simulink model "array_doubleRx"  (R2019b)
settings: Solver=VariableStepAuto  StartTime=0.0  StopTime=0.0005  RelTol=1e-3
libraries: fl_lib x109, nesl_utility x70, ee_lib x35, powerlib_meascontrol x11
settings Model: Creator=LRF  LastModifiedBy=LRF

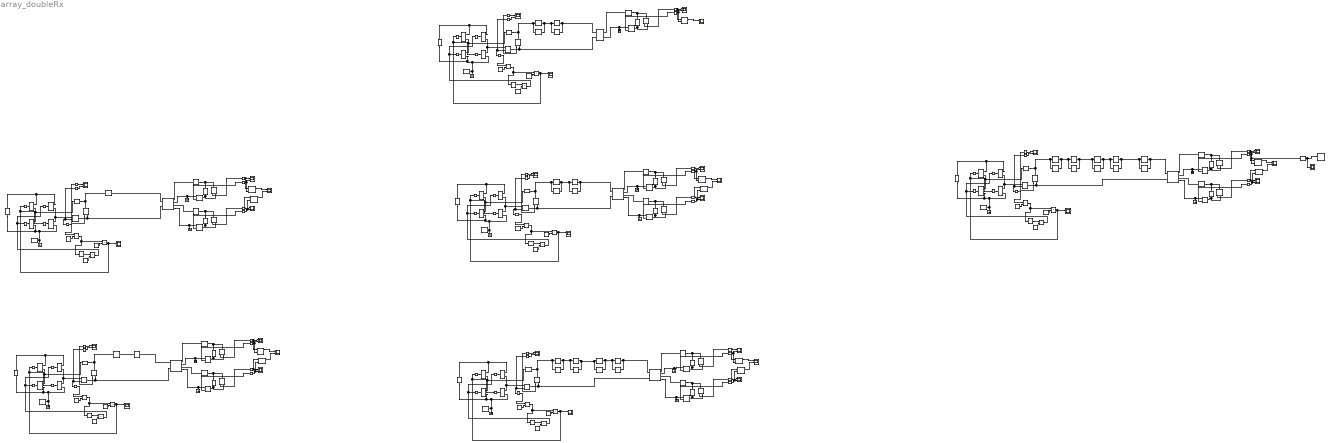
== system array_doubleRx ==
  (2/a-1)Ca{,1..12} (13 alike) : fl_lib/Electrical/Electrical Elements/Capacitor  c=379 pF  r=1e-6 Ohm  g=0 1/Ohm  i_specify=off  i_priority=None  i=0 A  i_nominal_specify=off  i_nominal_unit=A  i_nominal_value=1  v_specify=off  v_priority=None  v=0 V  v_nominal_specify=off  v_nominal_unit=V  v_nominal_value=1  vc_specify=off  vc_priority=High  vc=0 V  vc_nominal_specify=off  vc_nominal_unit=V  vc_nominal_value=1
  Ca{,1..15} (16 alike) : fl_lib/Electrical/Electrical Elements/Capacitor  c=1517 pF  r=1e-6 Ohm  g=0 1/Ohm  i_specify=off  i_priority=None  i=0 A  i_nominal_specify=off  i_nominal_unit=A  i_nominal_value=1  v_specify=off  v_priority=None  v=0 V  v_nominal_specify=off  v_nominal_unit=V  v_nominal_value=1  vc_specify=off  vc_priority=High  vc=0 V  vc_nominal_specify=off  vc_nominal_unit=V  vc_nominal_value=1
  Capacitor{1..10,12} (11 alike) : fl_lib/Electrical/Electrical Elements/Capacitor  c=1013 pF  r=1e-6 Ohm  g=0 1/Ohm  i_specify=off  i_priority=None  i=0 A  i_nominal_specify=off  i_nominal_unit=A  i_nominal_value=1  v_specify=off  v_priority=None  v=0 V  v_nominal_specify=off  v_nominal_unit=V  v_nominal_value=1  vc_specify=off  vc_priority=High  vc=0 V  vc_nominal_specify=off  vc_nominal_unit=V  vc_nominal_value=1
  Constant{,2,6,9,14..15} (6 alike) : Constant  Value=0
  Constant{1,3..5,7..8,10..13,16..17} (12 alike) : Constant  Value=12
  Current Sensor{,1..15,17} (17 alike) : fl_lib/Electrical/Electrical Sensors/Current Sensor
  Electrical Reference{,1..15,17} (17 alike) : fl_lib/Electrical/Electrical Elements/Electrical Reference
  GT{,1..5} (6 alike) : RelationalOperator  Operator=>  OutDataTypeStr=boolean  RndMeth=Simplest
  Logical Operator{,1..5} (6 alike) : Logic  Operator=NOT  AllPortsSameDT=off  OutDataTypeStr=boolean
  MOSFET (Ideal, Switching){,1..23} (24 alike) : ee_lib/Semiconductors & Converters/MOSFET (Ideal, Switching)  Rds=0.01 Ohm  Goff=1e-6 1/Ohm  Vth=2 V  diode_param=1  diode_Vf=0.8 V  diode_Ron=0.001 Ohm  diode_Goff=1e-5 1/Ohm  diode_C=50e-9 F  diode_iRM=-235 A  diode_iF=300 A  diode_idot=-50 A/us  diode_trr_param=1  diode_trr_factor=3  diode_trr=15 us  diode_Qrr=1500 s*uA  thermal_loss_option=2  Voff=300 V  Tau=1e-4 s  Tj=[298.15, 398.15] K  Iout_scalar=600 A  Eon_scalar=22.86e-3 J  Eoff_scalar=17.14e-3 J  Von_scalar=2.7 V  Iout_data=[0, 10, 50, 100, 200, 400, 600] A  Eon_data=[0, .29, 1.43, 2.86, 5.71, 13.14, 22.86; 0, .57, 2.63, 5.14, 10.29, 20.57, 30.29] * 1e-3 J  Eoff_data=[0, .21, 1.07, 2.14, 4.29, 9.86, 17.14; 0, .43, 1.97, 3.86, 7.71, 15.43, 22.71] * 1e-3 J  Von_data=[0, 1.1, 1.3, 1.45, 1.75, 2.25, 2.7; 0, 1, 1.15, 1.35, 1.7, 2.35, 3] V
      settings: SourceProductName=Simscape Electrical
  Mutual Inductor : fl_lib/Electrical/Electrical Elements/Mutual Inductor  L1=106.94 uH  L2=100 uH  k=0.1  i1_specify=off  i1_priority=High  i1=0 A  i1_nominal_specify=off  i1_nominal_unit=A  i1_nominal_value=1  i2_specify=off  i2_priority=High  i2=0 A  i2_nominal_specify=off  i2_nominal_unit=A  i2_nominal_value=1  v1_specify=off  v1_priority=None  v1=0 V  v1_nominal_specify=off  v1_nominal_unit=V  v1_nominal_value=1  v2_specify=off  v2_priority=None  v2=0 V  v2_nominal_specify=off  v2_nominal_unit=V  v2_nominal_value=1
      settings: SourceProductName=Simscape  SourceProductBaseCode=SS  InternalSimscapePortConfiguration="{\"Bottom\":[],\"Left\":[{\"id\":\"p1\",\"label\":\"1+\",\"type\":\"foundation.electrical.electrical\"},{\"id\":\"n1\",\"label\":\"1-\",\"type\":\"foundation.electrical.electrical\"}],\"Right\":[{\"id\":\"p2\",\"label\":\"2+\",\"type\":\"foundation.electrical.electrical\"},{\"id\":\"n2\",\"label\":\"2-\",\"type\":\"foundation.electrical.electrical\"}],\"Top\":[]}"
  PS-Simulink Converter{,1..37,40..41} (40 alike) : nesl_utility/PS-Simulink Converter  PhysicalDomain=network_engine_domain  SubClassName=ps_output  LeftPortType=input  RightPortType=output  PseudoPeriodic=off  Frequencies=[]  Unit=inherit  AffineConversion=off
  Power (Phasor){,1..9,11} (11 alike) : powerlib_meascontrol/Measurements/Power (Phasor)
      settings: SourceProductName=Simscape Electrical  SourceProductBaseCode=PS
  Product{,1..11} (12 alike) : Product
  Resistor{,3,6,9,14..15} (6 alike) : fl_lib/Electrical/Electrical Elements/Resistor  R=0 Ohm  i_specify=off  i_priority=None  i=0 A  i_nominal_specify=off  i_nominal_unit=A  i_nominal_value=1  v_specify=off  v_priority=None  v=0 V  v_nominal_specify=off  v_nominal_unit=V  v_nominal_value=1
  Resistor{1..2,4..5,7..8,10..13,17} (11 alike) : fl_lib/Electrical/Electrical Elements/Resistor  R=15 Ohm  i_specify=off  i_priority=None  i=0 A  i_nominal_specify=off  i_nominal_unit=A  i_nominal_value=1  v_specify=off  v_priority=None  v=0 V  v_nominal_specify=off  v_nominal_unit=V  v_nominal_value=1
  Scope{,1..24,26..27,29..30} (29 alike) : Scope  NumInputPorts=2
  Scope28 : Scope
  Simulink-PS Converter{,1..23} (24 alike) : nesl_utility/Simulink-PS Converter  PhysicalDomain=network_engine_domain  SubClassName=ps_input  LeftPortType=input  RightPortType=output  PseudoPeriodic=off  Frequencies=[]  NoiseDistribution=none  NoiseParameters=[]  Unit=1  AffineConversion=off  FilteringAndDerivatives=provide  SimscapeFilterOrder=1  InputFilterTimeConstant=0.001  UdotUserProvided=0
  Solver Configuration{,1..5} (6 alike) : nesl_utility/Solver Configuration  PhysicalDomain=network_engine_domain  SubClassName=solver  LeftPortType=input  RightPortType=generic  Tones=[]  Harmonics=[]  SimulateNoise=off  Profile=off  UseLocalSampling=off  EnableSwitchedLinearOptims=on  FrequencyDomain=off  UseCCode=off  RelTol=0.001  AbsTol=1e-06  MinStep=1e-09  ToWorkspace=off  RevertToSquareIcSolve=off  NumHomotopyIterations=100  PhasorMode=off  PhasorModeNumHarmonics=1  DoDC=off  ResidualTolerance=1e-09  UseLocalSolver=off  LocalSolverChoice=NE_BACKWARD_EULER_ADVANCER  LocalSolverSampleTime=0.001  DoFixedCost=off  MaxNonlinIter=3  MaxModeIter=2  LinearAlgebra=auto  EquationFormulation=NE_TIME_EF  DelaysMemoryBudget=1024  AutomaticFiltering=on  FilteringTimeConstant=0.001  PartitionStorageMethod=AS_NEEDED  PartitionMemoryBudget=1024  PartitionMethod=ROBUST
  Spectrum Analyzer2 : SpectrumAnalyzer
  Three-Winding Mutual Inductor : ee_lib/Passive/Transformers/Three-Winding Mutual Inductor  L1=106.94 uH  L2=100 uH  L3=100 uH  K12=0.1  K13=0.1  K23=0  IC_given=1  IC1=0 A  IC2=0 A  IC3=0 A
      settings: SourceProductName=Simscape Electrical  SourceProductBaseCode=PS  InternalSimscapePortConfiguration="{\"Bottom\":[],\"Left\":[{\"id\":\"p1\",\"label\":\"1+\",\"type\":\"foundation.electrical.electrical\"},{\"id\":\"n1\",\"label\":\"1-\",\"type\":\"foundation.electrical.electrical\"}],\"Right\":[{\"id\":\"p2\",\"label\":\"2+\",\"type\":\"foundation.electrical.electrical\"},{\"id\":\"n2\",\"label\":\"2-\",\"type\":\"foundation.electrical.electrical\"},{\"id\":\"p3\",\"label\":\"3+\",\"type\":\"foundation.electrical.electrical\"},{\"id\":\"n3\",\"label\":\"3-\",\"type\":\"foundation.electrical.electrical\"}],\"Top\":[]}"
  Three-Winding Mutual Inductor1 : ee_lib/Passive/Transformers/Three-Winding Mutual Inductor  L1=66.79 uH  L2=100 uH  L3=100 uH  K12=0.1  K13=0.1  K23=0  IC_given=1  IC1=0 A  IC2=0 A  IC3=0 A
      settings: SourceProductName=Simscape Electrical  SourceProductBaseCode=PS  InternalSimscapePortConfiguration="{\"Bottom\":[],\"Left\":[{\"id\":\"p1\",\"label\":\"1+\",\"type\":\"foundation.electrical.electrical\"},{\"id\":\"n1\",\"label\":\"1-\",\"type\":\"foundation.electrical.electrical\"}],\"Right\":[{\"id\":\"p2\",\"label\":\"2+\",\"type\":\"foundation.electrical.electrical\"},{\"id\":\"n2\",\"label\":\"2-\",\"type\":\"foundation.electrical.electrical\"},{\"id\":\"p3\",\"label\":\"3+\",\"type\":\"foundation.electrical.electrical\"},{\"id\":\"n3\",\"label\":\"3-\",\"type\":\"foundation.electrical.electrical\"}],\"Top\":[]}"
  Three-Winding Mutual Inductor2 : ee_lib/Passive/Transformers/Three-Winding Mutual Inductor  L1=133.58 uH  L2=100 uH  L3=100 uH  K12=0.1  K13=0.1  K23=0  IC_given=1  IC1=0 A  IC2=0 A  IC3=0 A
      settings: SourceProductName=Simscape Electrical  SourceProductBaseCode=PS  InternalSimscapePortConfiguration="{\"Bottom\":[],\"Left\":[{\"id\":\"p1\",\"label\":\"1+\",\"type\":\"foundation.electrical.electrical\"},{\"id\":\"n1\",\"label\":\"1-\",\"type\":\"foundation.electrical.electrical\"}],\"Right\":[{\"id\":\"p2\",\"label\":\"2+\",\"type\":\"foundation.electrical.electrical\"},{\"id\":\"n2\",\"label\":\"2-\",\"type\":\"foundation.electrical.electrical\"},{\"id\":\"p3\",\"label\":\"3+\",\"type\":\"foundation.electrical.electrical\"},{\"id\":\"n3\",\"label\":\"3-\",\"type\":\"foundation.electrical.electrical\"}],\"Top\":[]}"
  Three-Winding Mutual Inductor3 : ee_lib/Passive/Transformers/Three-Winding Mutual Inductor  L1=213.88 uH  L2=100 uH  L3=100 uH  K12=0.1  K13=0.1  K23=0  IC_given=1  IC1=0 A  IC2=0 A  IC3=0 A
      settings: SourceProductName=Simscape Electrical  SourceProductBaseCode=PS  InternalSimscapePortConfiguration="{\"Bottom\":[],\"Left\":[{\"id\":\"p1\",\"label\":\"1+\",\"type\":\"foundation.electrical.electrical\"},{\"id\":\"n1\",\"label\":\"1-\",\"type\":\"foundation.electrical.electrical\"}],\"Right\":[{\"id\":\"p2\",\"label\":\"2+\",\"type\":\"foundation.electrical.electrical\"},{\"id\":\"n2\",\"label\":\"2-\",\"type\":\"foundation.electrical.electrical\"},{\"id\":\"p3\",\"label\":\"3+\",\"type\":\"foundation.electrical.electrical\"},{\"id\":\"n3\",\"label\":\"3-\",\"type\":\"foundation.electrical.electrical\"}],\"Top\":[]}"
  Three-Winding Mutual Inductor4 : ee_lib/Passive/Transformers/Three-Winding Mutual Inductor  L1=280.67 uH  L2=100 uH  L3=100 uH  K12=0.1  K13=0.1  K23=0  IC_given=1  IC1=0 A  IC2=0 A  IC3=0 A
      settings: SourceProductName=Simscape Electrical  SourceProductBaseCode=PS  InternalSimscapePortConfiguration="{\"Bottom\":[],\"Left\":[{\"id\":\"p1\",\"label\":\"1+\",\"type\":\"foundation.electrical.electrical\"},{\"id\":\"n1\",\"label\":\"1-\",\"type\":\"foundation.electrical.electrical\"}],\"Right\":[{\"id\":\"p2\",\"label\":\"2+\",\"type\":\"foundation.electrical.electrical\"},{\"id\":\"n2\",\"label\":\"2-\",\"type\":\"foundation.electrical.electrical\"},{\"id\":\"p3\",\"label\":\"3+\",\"type\":\"foundation.electrical.electrical\"},{\"id\":\"n3\",\"label\":\"3-\",\"type\":\"foundation.electrical.electrical\"}],\"Top\":[]}"
  Voltage Sensor{,1..14,16..17} (17 alike) : fl_lib/Electrical/Electrical Sensors/Voltage Sensor
  Voltage Source : ee_lib/Sources/Voltage Source  dc_voltage=15 V  ac_voltage=0 V  ac_shift=0 rad  ac_frequency=60 Hz  noise_mode=0  PSD=0 V^2/Hz  repeatability=1  auto_seed=3646982598  user_seed=0  sample_time=1e-3 s  i_specify=off  i_priority=None  i=0 A  i_nominal_specify=off  i_nominal_unit=A  i_nominal_value=1  v_specify=off  v_priority=None  v=0 V  v_nominal_specify=off  v_nominal_unit=V  v_nominal_value=1
      settings: SourceProductName=Simscape Electrical
  Voltage Source1 : ee_lib/Sources/Voltage Source  dc_voltage=15 V  ac_voltage=0 V  ac_shift=0 rad  ac_frequency=60 Hz  noise_mode=0  PSD=0 V^2/Hz  repeatability=1  auto_seed=508128604  user_seed=0  sample_time=1e-3 s  i_specify=off  i_priority=None  i=0 A  i_nominal_specify=off  i_nominal_unit=A  i_nominal_value=1  v_specify=off  v_priority=None  v=0 V  v_nominal_specify=off  v_nominal_unit=V  v_nominal_value=1
      settings: SourceProductName=Simscape Electrical
  Voltage Source2 : ee_lib/Sources/Voltage Source  dc_voltage=15 V  ac_voltage=0 V  ac_shift=0 rad  ac_frequency=60 Hz  noise_mode=0  PSD=0 V^2/Hz  repeatability=1  auto_seed=746822400  user_seed=0  sample_time=1e-3 s  i_specify=off  i_priority=None  i=0 A  i_nominal_specify=off  i_nominal_unit=A  i_nominal_value=1  v_specify=off  v_priority=None  v=0 V  v_nominal_specify=off  v_nominal_unit=V  v_nominal_value=1
      settings: SourceProductName=Simscape Electrical
  Voltage Source3 : ee_lib/Sources/Voltage Source  dc_voltage=15 V  ac_voltage=0 V  ac_shift=0 rad  ac_frequency=60 Hz  noise_mode=0  PSD=0 V^2/Hz  repeatability=1  auto_seed=3181899151  user_seed=0  sample_time=1e-3 s  i_specify=off  i_priority=None  i=0 A  i_nominal_specify=off  i_nominal_unit=A  i_nominal_value=1  v_specify=off  v_priority=None  v=0 V  v_nominal_specify=off  v_nominal_unit=V  v_nominal_value=1
      settings: SourceProductName=Simscape Electrical
  Voltage Source4 : ee_lib/Sources/Voltage Source  dc_voltage=15 V  ac_voltage=0 V  ac_shift=0 rad  ac_frequency=60 Hz  noise_mode=0  PSD=0 V^2/Hz  repeatability=1  auto_seed=170723637  user_seed=0  sample_time=1e-3 s  i_specify=off  i_priority=None  i=0 A  i_nominal_specify=off  i_nominal_unit=A  i_nominal_value=1  v_specify=off  v_priority=None  v=0 V  v_nominal_specify=off  v_nominal_unit=V  v_nominal_value=1
      settings: SourceProductName=Simscape Electrical
  Voltage Source5 : ee_lib/Sources/Voltage Source  dc_voltage=15 V  ac_voltage=0 V  ac_shift=0 rad  ac_frequency=60 Hz  noise_mode=0  PSD=0 V^2/Hz  repeatability=1  auto_seed=2586388248  user_seed=0  sample_time=1e-3 s  i_specify=off  i_priority=None  i=0 A  i_nominal_specify=off  i_nominal_unit=A  i_nominal_value=1  v_specify=off  v_priority=None  v=0 V  v_nominal_specify=off  v_nominal_unit=V  v_nominal_value=1
      settings: SourceProductName=Simscape Electrical
  Zero-Order Hold1 : ZeroOrderHold  SampleTime=1e-7
  wires:
  PS-Simulink Converter/1 -> Scope/1
  PS-Simulink Converter2/1 -> Scope/2
  PS-Simulink Converter1/1 -> GT/1
  Constant/1 -> GT/2
  GT/1 -> Logical Operator/1, Product/1
  Product/1 -> Simulink-PS Converter3/1, Simulink-PS Converter1/1, Scope1/1
  Constant3/1 -> Product/2
  Logical Operator/1 -> Product1/1
  Constant1/1 -> Product1/2
  Product1/1 -> Simulink-PS Converter2/1, Simulink-PS Converter/1
  PS-Simulink Converter4/1 -> Power (Phasor)/2, Scope2/2
  PS-Simulink Converter3/1 -> Power (Phasor)/1, Scope2/1
  PS-Simulink Converter6/1 -> Power (Phasor)1/2, Scope3/2
  PS-Simulink Converter5/1 -> Power (Phasor)1/1, Scope3/1
  Power (Phasor)/1 -> Scope4/2
  Power (Phasor)1/1 -> Scope4/1
  PS-Simulink Converter7/1 -> Scope5/1
  PS-Simulink Converter9/1 -> Scope5/2
  PS-Simulink Converter8/1 -> GT1/1
  PS-Simulink Converter13/1 -> Power (Phasor)3/2, Scope8/2
  Power (Phasor)2/1 -> Scope9/2
  GT1/1 -> Logical Operator1/1, Product2/1
  PS-Simulink Converter10/1 -> Power (Phasor)2/1, Scope7/1
  Product2/1 -> Simulink-PS Converter7/1, Simulink-PS Converter5/1, Scope6/1
  Logical Operator1/1 -> Product3/1
  Product3/1 -> Simulink-PS Converter6/1, Simulink-PS Converter4/1
  Constant2/1 -> GT1/2
  PS-Simulink Converter11/1 -> Power (Phasor)2/2, Scope7/2
  Power (Phasor)3/1 -> Scope9/1
  Constant5/1 -> Product2/2
  Constant4/1 -> Product3/2
  PS-Simulink Converter12/1 -> Power (Phasor)3/1, Scope8/1
  Product5/1 -> Simulink-PS Converter10/1, Simulink-PS Converter8/1
  Logical Operator2/1 -> Product5/1
  GT2/1 -> Logical Operator2/1, Product4/1
  PS-Simulink Converter18/1 -> Scope10/1
  PS-Simulink Converter17/1 -> Power (Phasor)5/2, Scope13/2
  PS-Simulink Converter20/1 -> Scope10/2
  PS-Simulink Converter19/1 -> GT2/1
  Constant8/1 -> Product4/2
  Product4/1 -> Simulink-PS Converter11/1, Simulink-PS Converter9/1, Scope11/1
  PS-Simulink Converter16/1 -> Power (Phasor)5/1, Scope13/1
  PS-Simulink Converter15/1 -> Power (Phasor)4/2, Scope12/2
  PS-Simulink Converter14/1 -> Power (Phasor)4/1, Scope12/1
  Constant6/1 -> GT2/2
  Constant7/1 -> Product5/2
  Power (Phasor)5/1 -> Scope14/1
  Power (Phasor)4/1 -> Scope14/2
  PS-Simulink Converter21/1 -> Scope15/1
  PS-Simulink Converter23/1 -> Scope15/2
  PS-Simulink Converter22/1 -> GT3/1
  PS-Simulink Converter27/1 -> Power (Phasor)7/2, Scope18/2
  Power (Phasor)6/1 -> Scope19/2
  GT3/1 -> Logical Operator3/1, Product6/1
  PS-Simulink Converter24/1 -> Power (Phasor)6/1, Scope17/1
  Product6/1 -> Simulink-PS Converter15/1, Simulink-PS Converter13/1, Scope16/1
  Logical Operator3/1 -> Product7/1
  Product7/1 -> Simulink-PS Converter14/1, Simulink-PS Converter12/1
  Constant9/1 -> GT3/2
  PS-Simulink Converter25/1 -> Power (Phasor)6/2, Scope17/2
  Power (Phasor)7/1 -> Scope19/1
  Constant11/1 -> Product6/2
  Constant10/1 -> Product7/2
  PS-Simulink Converter26/1 -> Power (Phasor)7/1, Scope18/1
  PS-Simulink Converter33/1 -> Power (Phasor)9/1, Scope23/1
  PS-Simulink Converter32/1 -> Power (Phasor)8/2, Scope22/2
  Logical Operator4/1 -> Product9/1
  Constant13/1 -> Product8/2
  Product8/1 -> Simulink-PS Converter19/1, Simulink-PS Converter17/1, Scope21/1
  Product9/1 -> Simulink-PS Converter18/1, Simulink-PS Converter16/1
  Power (Phasor)9/1 -> Scope24/1
  PS-Simulink Converter31/1 -> Power (Phasor)8/1, Scope22/1
  Constant12/1 -> Product9/2
  Power (Phasor)8/1 -> Scope24/2
  GT4/1 -> Logical Operator4/1, Product8/1
  Constant14/1 -> GT4/2
  PS-Simulink Converter28/1 -> Scope20/1
  PS-Simulink Converter30/1 -> Scope20/2
  PS-Simulink Converter29/1 -> GT4/1
  PS-Simulink Converter35/1 -> Scope26/1
  PS-Simulink Converter37/1 -> Scope26/2
  PS-Simulink Converter36/1 -> GT5/1
  PS-Simulink Converter41/1 -> Power (Phasor)11/2, Scope29/2
  GT5/1 -> Logical Operator5/1, Product10/1
  Product10/1 -> Simulink-PS Converter23/1, Simulink-PS Converter21/1, Scope27/1
  Logical Operator5/1 -> Product11/1
  Product11/1 -> Simulink-PS Converter22/1, Simulink-PS Converter20/1
  Constant15/1 -> GT5/2
  Power (Phasor)11/1 -> Scope30/1
  Constant17/1 -> Product10/2
  Constant16/1 -> Product11/2
  PS-Simulink Converter40/1 -> Power (Phasor)11/1, Scope29/1
  Zero-Order Hold1/1 -> Scope28/1, Spectrum Analyzer2/1
  PS-Simulink Converter34/1 -> Zero-Order Hold1/1, Power (Phasor)9/2, Scope23/2
  connections:
  Electrical Reference1/LConn1 -- Three-Winding Mutual Inductor/RConn4 -- Current Sensor1/RConn2
  Capacitor1/RConn1 -- Voltage Sensor/LConn1 -- Resistor1/LConn1
  Capacitor1/LConn1 -- Three-Winding Mutual Inductor/RConn3
  Resistor/RConn1 -- (2/a-1)Ca/LConn1 -- Ca/LConn1 -- Voltage Sensor1/LConn1
  "MOSFET (Ideal, Switching)"/RConn1 -- Voltage Source/LConn1 -- "MOSFET (Ideal, Switching)2"/RConn1
  "MOSFET (Ideal, Switching)1"/RConn1 -- "MOSFET (Ideal, Switching)"/RConn2 -- Resistor/LConn1
  "MOSFET (Ideal, Switching)3"/RConn1 -- Current Sensor/RConn2 -- "MOSFET (Ideal, Switching)2"/RConn2
  "MOSFET (Ideal, Switching)1"/RConn2 -- Voltage Source/RConn1 -- Solver Configuration/RConn1 -- Electrical Reference/LConn1 -- "MOSFET (Ideal, Switching)3"/RConn2
  Simulink-PS Converter/RConn1 -- "MOSFET (Ideal, Switching)1"/LConn1
  Simulink-PS Converter1/RConn1 -- "MOSFET (Ideal, Switching)"/LConn1
  Simulink-PS Converter2/RConn1 -- "MOSFET (Ideal, Switching)2"/LConn1
  Simulink-PS Converter3/RConn1 -- "MOSFET (Ideal, Switching)3"/LConn1
  Voltage Sensor1/RConn2 -- Three-Winding Mutual Inductor/LConn2 -- Current Sensor/LConn1
  Current Sensor/RConn1 -- PS-Simulink Converter2/LConn1 -- PS-Simulink Converter1/LConn1
  Voltage Sensor/RConn2 -- Current Sensor1/LConn1 -- Resistor1/RConn1
  Voltage Sensor1/RConn1 -- PS-Simulink Converter/LConn1
  PS-Simulink Converter3/LConn1 -- Voltage Sensor/RConn1
  Current Sensor1/RConn1 -- PS-Simulink Converter4/LConn1
  Resistor2/RConn1 -- Voltage Sensor2/RConn2 -- Current Sensor2/LConn1
  Current Sensor2/RConn2 -- Electrical Reference2/LConn1 -- Three-Winding Mutual Inductor/RConn2
  Resistor2/LConn1 -- Capacitor3/RConn1 -- Voltage Sensor2/LConn1
  Capacitor3/LConn1 -- Three-Winding Mutual Inductor/RConn1
  PS-Simulink Converter5/LConn1 -- Voltage Sensor2/RConn1
  Current Sensor2/RConn1 -- PS-Simulink Converter6/LConn1
  (2/a-1)Ca/RConn1 -- (2/a-1)Ca1/LConn1 -- Ca1/LConn1 -- Ca/RConn1
  (2/a-1)Ca1/RConn1 -- Three-Winding Mutual Inductor/LConn1 -- Ca1/RConn1
  Current Sensor4/RConn2 -- Electrical Reference4/LConn1 -- Three-Winding Mutual Inductor1/RConn4
  Three-Winding Mutual Inductor1/RConn2 -- Current Sensor5/RConn2 -- Electrical Reference5/LConn1
  Resistor4/LConn1 -- Capacitor2/RConn1 -- Voltage Sensor3/LConn1
  Voltage Sensor4/LConn1 -- Resistor3/RConn1 -- Ca2/LConn1
  Current Sensor5/LConn1 -- Resistor5/RConn1 -- Voltage Sensor5/RConn2
  "MOSFET (Ideal, Switching)6"/RConn1 -- "MOSFET (Ideal, Switching)4"/RConn1 -- Voltage Source1/LConn1
  "MOSFET (Ideal, Switching)6"/RConn2 -- "MOSFET (Ideal, Switching)7"/RConn1 -- Current Sensor3/RConn2
  Three-Winding Mutual Inductor1/LConn1 -- Ca2/RConn1
  Resistor3/LConn1 -- "MOSFET (Ideal, Switching)5"/RConn1 -- "MOSFET (Ideal, Switching)4"/RConn2
  PS-Simulink Converter8/LConn1 -- Current Sensor3/RConn1 -- PS-Simulink Converter9/LConn1
  Voltage Sensor5/LConn1 -- Resistor5/LConn1 -- Capacitor4/RConn1
  Current Sensor3/LConn1 -- Voltage Sensor4/RConn2 -- Three-Winding Mutual Inductor1/LConn2
  "MOSFET (Ideal, Switching)7"/RConn2 -- Solver Configuration1/RConn1 -- Electrical Reference3/LConn1 -- "MOSFET (Ideal, Switching)5"/RConn2 -- Voltage Source1/RConn1
  Resistor4/RConn1 -- Voltage Sensor3/RConn2 -- Current Sensor4/LConn1
  Capacitor4/LConn1 -- Three-Winding Mutual Inductor1/RConn1
  PS-Simulink Converter12/LConn1 -- Voltage Sensor5/RConn1
  Simulink-PS Converter5/RConn1 -- "MOSFET (Ideal, Switching)4"/LConn1
  Simulink-PS Converter4/RConn1 -- "MOSFET (Ideal, Switching)5"/LConn1
  Current Sensor4/RConn1 -- PS-Simulink Converter11/LConn1
  Simulink-PS Converter7/RConn1 -- "MOSFET (Ideal, Switching)7"/LConn1
  Simulink-PS Converter6/RConn1 -- "MOSFET (Ideal, Switching)6"/LConn1
  Current Sensor5/RConn1 -- PS-Simulink Converter13/LConn1
  Voltage Sensor4/RConn1 -- PS-Simulink Converter7/LConn1
  Capacitor2/LConn1 -- Three-Winding Mutual Inductor1/RConn3
  PS-Simulink Converter10/LConn1 -- Voltage Sensor3/RConn1
  Resistor7/RConn1 -- Voltage Sensor6/RConn2 -- Current Sensor7/LConn1
  "MOSFET (Ideal, Switching)10"/RConn1 -- "MOSFET (Ideal, Switching)8"/RConn1 -- Voltage Source2/LConn1
  Current Sensor6/LConn1 -- Voltage Sensor7/RConn2 -- Three-Winding Mutual Inductor2/LConn2
  Voltage Sensor7/LConn1 -- Resistor6/RConn1 -- Ca3/LConn1
  Resistor7/LConn1 -- Capacitor5/RConn1 -- Voltage Sensor6/LConn1
  Voltage Source2/RConn1 -- "MOSFET (Ideal, Switching)9"/RConn2 -- Solver Configuration2/RConn1 -- Electrical Reference6/LConn1 -- "MOSFET (Ideal, Switching)11"/RConn2
  Current Sensor7/RConn2 -- Electrical Reference7/LConn1 -- Three-Winding Mutual Inductor2/RConn4
  Resistor6/LConn1 -- "MOSFET (Ideal, Switching)9"/RConn1 -- "MOSFET (Ideal, Switching)8"/RConn2
  Three-Winding Mutual Inductor2/RConn2 -- Current Sensor8/RConn2 -- Electrical Reference8/LConn1
  Current Sensor8/LConn1 -- Resistor8/RConn1 -- Voltage Sensor8/RConn2
  PS-Simulink Converter19/LConn1 -- Current Sensor6/RConn1 -- PS-Simulink Converter20/LConn1
  Voltage Sensor8/LConn1 -- Resistor8/LConn1 -- Capacitor6/RConn1
  "MOSFET (Ideal, Switching)10"/RConn2 -- "MOSFET (Ideal, Switching)11"/RConn1 -- Current Sensor6/RConn2
  Simulink-PS Converter10/RConn1 -- "MOSFET (Ideal, Switching)10"/LConn1
  Voltage Sensor7/RConn1 -- PS-Simulink Converter18/LConn1
  Capacitor5/LConn1 -- Three-Winding Mutual Inductor2/RConn3
  Simulink-PS Converter11/RConn1 -- "MOSFET (Ideal, Switching)11"/LConn1
  Current Sensor8/RConn1 -- PS-Simulink Converter17/LConn1
  PS-Simulink Converter16/LConn1 -- Voltage Sensor8/RConn1
  Capacitor6/LConn1 -- Three-Winding Mutual Inductor2/RConn1
  Current Sensor7/RConn1 -- PS-Simulink Converter15/LConn1
  PS-Simulink Converter14/LConn1 -- Voltage Sensor6/RConn1
  Simulink-PS Converter9/RConn1 -- "MOSFET (Ideal, Switching)8"/LConn1
  Simulink-PS Converter8/RConn1 -- "MOSFET (Ideal, Switching)9"/LConn1
  Three-Winding Mutual Inductor2/LConn1 -- Ca4/RConn1
  Ca4/LConn1 -- Ca3/RConn1
  (2/a-1)Ca4/LConn1 -- Ca7/LConn1 -- Ca6/RConn1 -- (2/a-1)Ca3/RConn1
  Current Sensor10/RConn2 -- Electrical Reference10/LConn1 -- Three-Winding Mutual Inductor3/RConn4
  Three-Winding Mutual Inductor3/RConn2 -- Current Sensor11/RConn2 -- Electrical Reference11/LConn1
  Resistor10/LConn1 -- Capacitor7/RConn1 -- Voltage Sensor9/LConn1
  Voltage Sensor10/LConn1 -- Resistor9/RConn1 -- (2/a-1)Ca2/LConn1 -- Ca5/LConn1
  Current Sensor11/LConn1 -- Resistor11/RConn1 -- Voltage Sensor11/RConn2
  "MOSFET (Ideal, Switching)14"/RConn1 -- "MOSFET (Ideal, Switching)12"/RConn1 -- Voltage Source3/LConn1
  "MOSFET (Ideal, Switching)14"/RConn2 -- "MOSFET (Ideal, Switching)15"/RConn1 -- Current Sensor9/RConn2
  Ca5/RConn1 -- (2/a-1)Ca2/RConn1 -- (2/a-1)Ca3/LConn1 -- Ca6/LConn1
  Resistor9/LConn1 -- "MOSFET (Ideal, Switching)13"/RConn1 -- "MOSFET (Ideal, Switching)12"/RConn2
  PS-Simulink Converter22/LConn1 -- Current Sensor9/RConn1 -- PS-Simulink Converter23/LConn1
  Voltage Sensor11/LConn1 -- Resistor11/LConn1 -- Capacitor8/RConn1
  Current Sensor9/LConn1 -- Voltage Sensor10/RConn2 -- Three-Winding Mutual Inductor3/LConn2
  "MOSFET (Ideal, Switching)15"/RConn2 -- Solver Configuration3/RConn1 -- Electrical Reference9/LConn1 -- "MOSFET (Ideal, Switching)13"/RConn2 -- Voltage Source3/RConn1
  Resistor10/RConn1 -- Voltage Sensor9/RConn2 -- Current Sensor10/LConn1
  Capacitor8/LConn1 -- Three-Winding Mutual Inductor3/RConn1
  PS-Simulink Converter26/LConn1 -- Voltage Sensor11/RConn1
  Simulink-PS Converter13/RConn1 -- "MOSFET (Ideal, Switching)12"/LConn1
  Capacitor7/LConn1 -- Three-Winding Mutual Inductor3/RConn3
  Current Sensor10/RConn1 -- PS-Simulink Converter25/LConn1
  Simulink-PS Converter15/RConn1 -- "MOSFET (Ideal, Switching)15"/LConn1
  Simulink-PS Converter14/RConn1 -- "MOSFET (Ideal, Switching)14"/LConn1
  Current Sensor11/RConn1 -- PS-Simulink Converter27/LConn1
  PS-Simulink Converter24/LConn1 -- Voltage Sensor9/RConn1
  Voltage Sensor10/RConn1 -- PS-Simulink Converter21/LConn1
  Simulink-PS Converter12/RConn1 -- "MOSFET (Ideal, Switching)13"/LConn1
  Ca8/LConn1 -- (2/a-1)Ca5/LConn1 -- (2/a-1)Ca4/RConn1 -- Ca7/RConn1
  (2/a-1)Ca5/RConn1 -- Three-Winding Mutual Inductor3/LConn1 -- Ca8/RConn1
  Voltage Sensor12/LConn1 -- Resistor14/RConn1 -- (2/a-1)Ca6/LConn1 -- Ca9/LConn1
  Resistor12/RConn1 -- Voltage Sensor14/RConn2 -- Current Sensor12/LConn1
  "MOSFET (Ideal, Switching)19"/RConn2 -- Solver Configuration4/RConn1 -- Electrical Reference14/LConn1 -- "MOSFET (Ideal, Switching)17"/RConn2 -- Voltage Source4/RConn1
  Current Sensor14/LConn1 -- Voltage Sensor12/RConn2 -- Three-Winding Mutual Inductor4/LConn2
  Resistor12/LConn1 -- Capacitor9/RConn1 -- Voltage Sensor14/LConn1
  Voltage Sensor13/LConn1 -- Resistor13/LConn1 -- Capacitor10/RConn1
  "MOSFET (Ideal, Switching)18"/RConn1 -- "MOSFET (Ideal, Switching)16"/RConn1 -- Voltage Source4/LConn1
  Ca10/LConn1 -- (2/a-1)Ca7/LConn1 -- (2/a-1)Ca6/RConn1 -- Ca9/RConn1
  Three-Winding Mutual Inductor4/RConn2 -- Current Sensor13/RConn2 -- Electrical Reference13/LConn1
  Resistor14/LConn1 -- "MOSFET (Ideal, Switching)17"/RConn1 -- "MOSFET (Ideal, Switching)16"/RConn2
  Ca12/LConn1 -- (2/a-1)Ca9/LConn1 -- (2/a-1)Ca8/RConn1 -- Ca11/RConn1
  Current Sensor12/RConn2 -- Electrical Reference12/LConn1 -- Three-Winding Mutual Inductor4/RConn4
  Current Sensor13/LConn1 -- Resistor13/RConn1 -- Voltage Sensor13/RConn2
  PS-Simulink Converter29/LConn1 -- Current Sensor14/RConn1 -- PS-Simulink Converter30/LConn1
  (2/a-1)Ca10/LConn1 -- Ca12/RConn1 -- (2/a-1)Ca9/RConn1 -- Ca13/LConn1
  (2/a-1)Ca7/RConn1 -- Ca11/LConn1 -- (2/a-1)Ca8/LConn1 -- Ca10/RConn1
  "MOSFET (Ideal, Switching)18"/RConn2 -- "MOSFET (Ideal, Switching)19"/RConn1 -- Current Sensor14/RConn2
  PS-Simulink Converter33/LConn1 -- Voltage Sensor13/RConn1
  Voltage Sensor12/RConn1 -- PS-Simulink Converter28/LConn1
  Capacitor9/LConn1 -- Three-Winding Mutual Inductor4/RConn3
  Current Sensor12/RConn1 -- PS-Simulink Converter32/LConn1
  Capacitor10/LConn1 -- Three-Winding Mutual Inductor4/RConn1
  Current Sensor13/RConn1 -- PS-Simulink Converter34/LConn1
  Simulink-PS Converter18/RConn1 -- "MOSFET (Ideal, Switching)18"/LConn1
  Simulink-PS Converter16/RConn1 -- "MOSFET (Ideal, Switching)17"/LConn1
  PS-Simulink Converter31/LConn1 -- Voltage Sensor14/RConn1
  Simulink-PS Converter19/RConn1 -- "MOSFET (Ideal, Switching)19"/LConn1
  Simulink-PS Converter17/RConn1 -- "MOSFET (Ideal, Switching)16"/LConn1
  (2/a-1)Ca10/RConn1 -- Ca13/RConn1 -- Three-Winding Mutual Inductor4/LConn1
  Ca15/RConn1 -- Mutual Inductor/LConn1 -- (2/a-1)Ca12/RConn1
  Electrical Reference17/LConn1 -- Mutual Inductor/RConn2 -- Current Sensor17/RConn2
  Voltage Sensor16/LConn1 -- Resistor15/RConn1 -- (2/a-1)Ca11/LConn1 -- Ca14/LConn1
  Current Sensor17/LConn1 -- Resistor17/RConn1 -- Voltage Sensor17/RConn2
  "MOSFET (Ideal, Switching)22"/RConn1 -- "MOSFET (Ideal, Switching)20"/RConn1 -- Voltage Source5/LConn1
  "MOSFET (Ideal, Switching)22"/RConn2 -- "MOSFET (Ideal, Switching)23"/RConn1 -- Current Sensor15/RConn2
  Ca14/RConn1 -- (2/a-1)Ca11/RConn1 -- (2/a-1)Ca12/LConn1 -- Ca15/LConn1
  Resistor15/LConn1 -- "MOSFET (Ideal, Switching)21"/RConn1 -- "MOSFET (Ideal, Switching)20"/RConn2
  PS-Simulink Converter36/LConn1 -- Current Sensor15/RConn1 -- PS-Simulink Converter37/LConn1
  Voltage Sensor17/LConn1 -- Resistor17/LConn1 -- Capacitor12/RConn1
  Current Sensor15/LConn1 -- Mutual Inductor/LConn2 -- Voltage Sensor16/RConn2
  "MOSFET (Ideal, Switching)23"/RConn2 -- Solver Configuration5/RConn1 -- Electrical Reference15/LConn1 -- "MOSFET (Ideal, Switching)21"/RConn2 -- Voltage Source5/RConn1
  Capacitor12/LConn1 -- Mutual Inductor/RConn1
  PS-Simulink Converter40/LConn1 -- Voltage Sensor17/RConn1
  Simulink-PS Converter21/RConn1 -- "MOSFET (Ideal, Switching)20"/LConn1
  Simulink-PS Converter20/RConn1 -- "MOSFET (Ideal, Switching)21"/LConn1
  Simulink-PS Converter23/RConn1 -- "MOSFET (Ideal, Switching)23"/LConn1
  Simulink-PS Converter22/RConn1 -- "MOSFET (Ideal, Switching)22"/LConn1
  Voltage Sensor16/RConn1 -- PS-Simulink Converter35/LConn1
  Current Sensor17/RConn1 -- PS-Simulink Converter41/LConn1
